simulink model "Wifi_IO"  (R2020b)
settings: Solver=VariableStepAuto  StartTime=0.0  StopTime=10.0  RelTol=1e-3
libraries: arduinomotorcarrierlib x2, arduinowifilib x2, eePwmGenerator x1
settings Model: Creator=gbellido  LastModifiedBy=gbellido

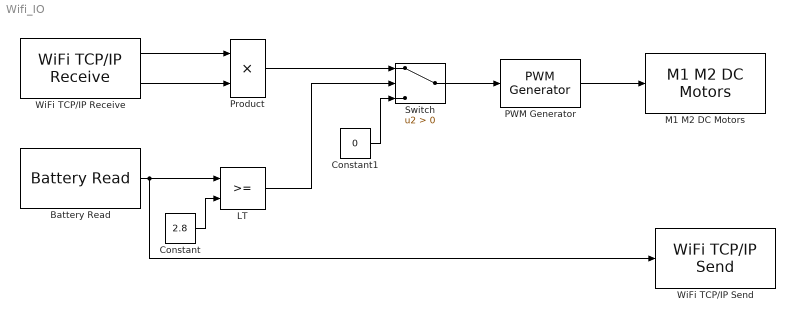
== system Wifi_IO ==
  Battery Read : arduinomotorcarrierlib/Battery Read  SlaveAddress=uint8( hex2dec( '66' ) )  blockPlatform=ARDUINO  SampleTime=0.1
      settings: SourceProductBaseCode=ARDUINO
  Constant : Constant  Value=2.8
  Constant1 : Constant  Value=0
  LT : RelationalOperator  OutDataTypeStr=boolean  RndMeth=Simplest
  M1 M2 DC Motors : arduinomotorcarrierlib/M1 M2 DC Motors  SlaveAddress=uint8( hex2dec( '66' ) )  blockPlatform=ARDUINO  MotorNumber=M1  MotorCarrierPWMFreq=100
      settings: SourceProductBaseCode=ARDUINO
  PWM Generator : eePwmGenerator/PWM Generator  CarrCount=Up  Tper=0.001  Ts=5e-5
  Product : Product
  Switch : Switch  Criteria=u2 > Threshold
  WiFi TCP/IP Receive : arduinowifilib/WiFi TCP//IP Receive  Mode_=Server  serverport=25000  RemoteAddr_=192.168.1.2  RemoteServerPort_=25000  DataType_=uint8  DataSize_=1  SampleTime_=0.1  remoteipoctet1=192  remoteipoctet2=168  remoteipoctet3=1  remoteipoctet4=2  wifiTCPServerIndex=0  wifiTCPClientIndex=0  blockPlatform=ARDUINO  isARMArch=false  SimulateUsing=Code generation  BlockingMode_=off  BlockTimeout_=0.1
      settings: SourceProductBaseCode=ARDUINO
  WiFi TCP/IP Send : arduinowifilib/WiFi TCP//IP Send  Mode_=Server  serverport=25000  RemoteAddr_=192.168.1.2  RemoteServerPort_=25000  remoteipoctet1=192  remoteipoctet2=168  remoteipoctet3=1  remoteipoctet4=2  wifiTCPServerIndex=0  wifiTCPClientIndex=0  blockPlatform=ARDUINO  isARMArch=false  SimulateUsing=Code generation
      settings: SourceProductBaseCode=ARDUINO
  wires:
  WiFi TCP/IP Receive/1 -> Product/1
  WiFi TCP/IP Receive/2 -> Product/2
  Battery Read/1 -> LT/1, WiFi TCP/IP Send/1
  Constant/1 -> LT/2
  LT/1 -> Switch/2
  Switch/1 -> PWM Generator/1
  Product/1 -> Switch/1
  Constant1/1 -> Switch/3
  PWM Generator/1 -> M1 M2 DC Motors/1
